simulink model "GE275103"  (R2015b)
settings: Solver=ode4  StartTime=0.0  StopTime=30  FixedStep=5e-6  RelTol=1e-3
PreLoadFcn:
  | Ts=5e-6;
values from neighbouring files (symbols this model uses):
  Cdc = 27e-3    (= 0.027)    [GE275103.m]    (also in GEWT.m)
  gear = 97    [GEWT.m]
  Jtotal = Jgen+Jtur/(gear^2)    (= 1581.65586141)    [GEWT.m]
  Ld = 10e-4    (= 0.001)    [GE275103.m]    (also in GEWT.m = 0.000248)
  Lfilter = 2e-4    (= 0.0002)    [GE275103.m]
  Lq = 10.5e-4    (= 0.00105)    [GE275103.m]    (also in GEWT.m = 0.000292)
  p = 1.225    [GE275103.m]    (also in GEWT.m)
  pgen = 2    [GE275103.m]    (also in GEWT.m = 4)
  Prated = 2750000    [GE275103.m]    (also in GEWT.m)
  R = 51.5    [GEWT.m]
  Rs = 1e-10    [GE275103.m]    (also in GEWT.m = 0.0007305)
  Vdcset = 2500    [GE275103.m]    (also in GEWT.m = 1100)
  windspeed = 10    [GEWT.m]
  winit = -160    [GEWT.m]
libraries: powerlib x17, powerlib_meascontrol x14, simulink x7
Description:
  | Copyright 2008-2013 The MathWorks, Inc.
settings Model: FPTRunName=Active  NumberOfSteps=800000  ExtModeAutoUpdateStatusClock=off  Creator=MathWorks  LastModifiedBy=Eren
settings DataIOCC: SaveFormat=Array  SignalLoggingSaveFormat=ModelDataLogs  SaveOutput=off  SignalLogging=off  SaveTime=off  SignalLoggingName=sigsOut
settings OptimizationCC: BlockReduction=off  BooleanDataType=off  ExpressionDepthLimit=2147483647  InitFltsAndDblsToZero=on
settings DebuggingCC: UnderspecifiedInitializationDetection=Classic  MergeDetectMultiDrivingBlocksExec=none  CheckExecutionContextPreStartOutputMsg=on  CheckExecutionContextRuntimeOutputMsg=on  SignalResolutionControl=TryResolveAllWithWarning  MultiTaskDSMMsg=warning  MultiTaskCondExecSysMsg=none  FcnCallInpInsideContextMsg=UseLocalSettings  StateNameClashWarn=warning
settings HardwareCC: ProdBitPerPointer=32  ProdLargestAtomicFloat=None  ProdIntDivRoundTo=Undefined  ProdEndianess=Unspecified  ProdWordSize=32  ProdHWDeviceType=32-bit Generic  TargetBitPerPointer=64  TargetLongLongMode=on  TargetIntDivRoundTo=Zero  TargetEndianess=LittleEndian  TargetWordSize=64  TargetHWDeviceType=MATLAB Host
settings GRTTargetCC: GeneratePreprocessorConditionals=Disable all  CombineOutputUpdateFcns=off  GRTInterface=on
settings ConfigComp: CovModelRefEnable=Off

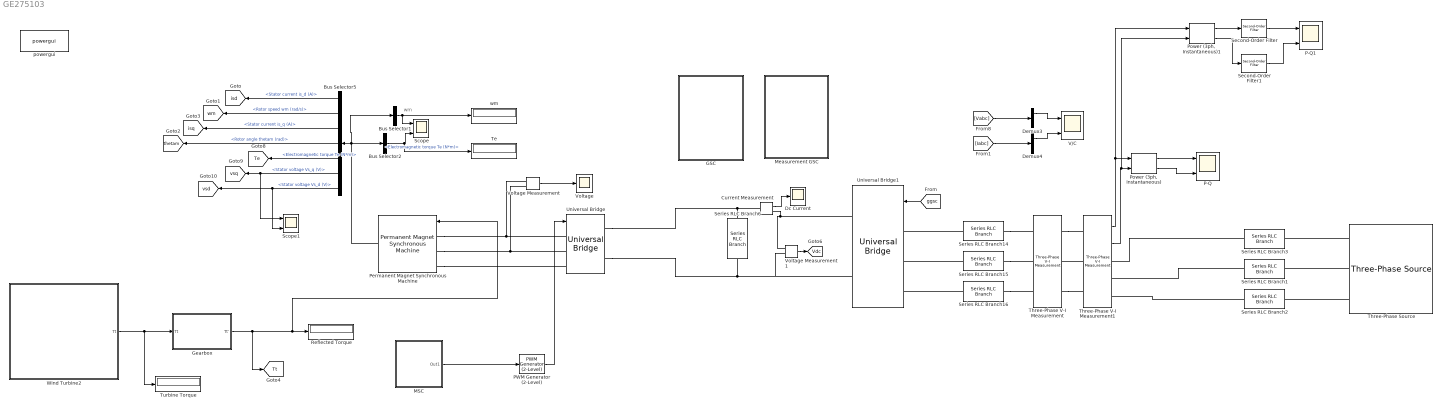
== system GE275103 ==
  note: wm
  Bus Selector1 : BusSelector  OutputSignals=Rotor speed wm (rad/s)  OutputAsBus=on
  Bus Selector2 : BusSelector  OutputSignals=Electromagnetic torque Te (N*m)
  Bus Selector5 : BusSelector  OutputSignals=Stator current is_d (A),Rotor speed wm (rad/s),Stator current is_q (A),Rotor angle thetam (rad),Electromagnetic torque Te (N*m),Stator voltage Vs_q (V),Stator voltage Vs_d (V)
  Current Measurement : powerlib/Measurements/Current Measurement  PhasorSimulation=off  OutputType=Complex  PSBequivalent=0
  Dc Current : Scope
  Demux3 : Demux  Outputs=3
  Demux4 : Demux  Outputs=3
  GSC : Subsystem
  Gearbox : Subsystem
  MSC : Subsystem
  Measurement GSC : Subsystem
  P-Q : Scope  NumInputPorts=2
  P-Q1 : Scope  NumInputPorts=2
  PWM Generator (2-Level) : powerlib_meascontrol/Pulse & Signal Generators/PWM Generator (2-Level)  ModulatorType=Three-phase bridge (6 pulses)  ModulatorMode=Unsynchronized  Fc=drivefreq  Pc=90  nF=60  MinMax="[ -1  1 ]"  SamplingTechnique=Natural  ModulatingSignals=off  m=0.8  Freq=60  Phase=0  Ts=Ts  ShowCarrierOutport=off
  Permanent Magnet Synchronous Machine : powerlib/Machines/Permanent Magnet Synchronous Machine  NbPhases=3  FluxDistribution=Sinusoidal  RotorType=Salient-pole  MechanicalLoad=Torque Tm  PresetModel=No  ShowDetailedParameters=on  MeasurementBus=off  Resistance=Rs  Inductance=8.5e-3  dqInductances=[Ld,Lq]  La=Lq  MachineConstant=Flux linkage established by magnets (V.s)  Flux=fluxlinkage  VoltageCst=1451.0395  TorqueCst=12  Flat=120  Mechanical=[Jtotal 1.349e-05 pgen 0]  PolePairs=2  InitialConditions=[winit,0, 0,0]  InitialConditions5ph=[0 0 0 0 0 0]  TsPowergui=0  TsBlock=-1  RefAngle=Aligned with phase A axis (original Park)
  "Power (3ph, Instantaneous)" : powerlib_meascontrol/Measurements/Power (3ph, Instantaneous)
  "Power (3ph, Instantaneous)1" : powerlib_meascontrol/Measurements/Power (3ph, Instantaneous)
  Reflected Torque : Display
  Scope : Scope  NumInputPorts=2
  Scope1 : Scope  NumInputPorts=2
  Second-Order Filter : powerlib_meascontrol/Filters/Second-Order Filter  FilterType=Lowpass  Fo=20  Zeta=0.707  Ts=0  Initialize=off  Vac_Init="[0,  0,  60]"  Vdc_Init=0  PlotResponse=off  FreqRange=[0, 500, 1]
  Second-Order Filter1 : powerlib_meascontrol/Filters/Second-Order Filter  FilterType=Lowpass  Fo=120  Zeta=0.707  Ts=0  Initialize=off  Vac_Init="[0,  0,  60]"  Vdc_Init=0  PlotResponse=off  FreqRange=[0, 500, 1]
  Series RLC Branch1 : powerlib/Elements/Series RLC Branch  LConnTagsString=__new0  RConnTagsString=__new0  BranchType=R  Resistance=0.001  Inductance=1e-3  SetiL0=off  InitialCurrent=0  Capacitance=1e-6  Setx0=off  InitialVoltage=0  Measurements=None
  Series RLC Branch14 : powerlib/Elements/Series RLC Branch  LConnTagsString=__new0  RConnTagsString=__new0  BranchType=L  Resistance=1  Inductance=Lfilter  SetiL0=off  InitialCurrent=0  Capacitance=1e-6  Setx0=off  InitialVoltage=0  Measurements=None
  Series RLC Branch15 : powerlib/Elements/Series RLC Branch  LConnTagsString=__new0  RConnTagsString=__new0  BranchType=L  Resistance=1  Inductance=Lfilter  SetiL0=off  InitialCurrent=0  Capacitance=1e-6  Setx0=off  InitialVoltage=0  Measurements=None
  Series RLC Branch16 : powerlib/Elements/Series RLC Branch  LConnTagsString=__new0  RConnTagsString=__new0  BranchType=L  Resistance=1  Inductance=Lfilter  SetiL0=off  InitialCurrent=0  Capacitance=1e-6  Setx0=off  InitialVoltage=0  Measurements=None
  Series RLC Branch2 : powerlib/Elements/Series RLC Branch  LConnTagsString=__new0  RConnTagsString=__new0  BranchType=R  Resistance=0.001  Inductance=1e-3  SetiL0=off  InitialCurrent=0  Capacitance=1e-6  Setx0=off  InitialVoltage=0  Measurements=None
  Series RLC Branch3 : powerlib/Elements/Series RLC Branch  LConnTagsString=__new0  RConnTagsString=__new0  BranchType=R  Resistance=0.001  Inductance=1e-3  SetiL0=off  InitialCurrent=0  Capacitance=1e-6  Setx0=off  InitialVoltage=0  Measurements=None
  Series RLC Branch6 : powerlib/Elements/Series RLC Branch  LConnTagsString=__new0  RConnTagsString=__new0  BranchType=C  Resistance=1  Inductance=1e-4  SetiL0=off  InitialCurrent=0  Capacitance=Cdc  Setx0=off  InitialVoltage=0  Measurements=None
  Te : Display
  Three-Phase V-I Measurement : powerlib/Measurements/Three-Phase V-I Measurement  VoltageMeasurement=phase-to-ground  SetLabelV=on  LabelV=Vabc  Vpu=on  VpuLL=off  CurrentMeasurement=yes  SetLabelI=on  LabelI=Iabc  Ipu=on  Pbase=2.75e6  Vbase=690  OutputType=Complex  PhasorSimulation=off  PSBequivalent=0
  Three-Phase V-I Measurement1 : powerlib/Measurements/Three-Phase V-I Measurement  VoltageMeasurement=phase-to-ground  SetLabelV=off  LabelV=Vabc  Vpu=off  VpuLL=off  CurrentMeasurement=yes  SetLabelI=off  LabelI=Iabc  Ipu=off  Pbase=2.75e6  Vbase=690  OutputType=Complex  PhasorSimulation=off  PSBequivalent=0
  Three-Phase Source : powerlib/Electrical Sources/Three-Phase Source  InternalConnection=Yg  VoltagePhases=off  Voltage=690  PhaseAngle=0  Voltage_phases=[25e3 25e3 25e3]/sqrt(3)  PhaseAngles_phases=[0 -120 +120]  Frequency=50  NonIdealSource=on  SpecifyImpedance=off  Resistance=0  Inductance=0  ShortCircuitLevel=100e6  BaseVoltage=690  XRratio=7  BusType=swing  Pref=10e3  Qref=0  Prefabc=[10e3, 10e3, 10e3]  Qrefabc=[0, 0, 0]  Qmin=-inf  Qmax=inf
  Turbine Torque : Display
  Universal Bridge : powerlib/Power Electronics/Universal Bridge  Arms=3  SnubberResistance=1e5  SnubberCapacitance=inf  Device=IGBT / Diodes  Ron=1e-3  Lon=0  ForwardVoltages="[  0  0  ]"  ForwardVoltage=0  GTOparameters=[ 10e-6 , 20e-6 ]  IGBTparameters=[ 1e-6 , 2e-6 ]  Measurements=None  Measurements_2=None  converterType=Rectifier
  Universal Bridge1 : powerlib/Power Electronics/Universal Bridge  Arms=3  SnubberResistance=1e5  SnubberCapacitance=inf  Device=IGBT / Diodes  Ron=0.00001  Lon=0  ForwardVoltages="[  0  0  ]"  ForwardVoltage=0  GTOparameters=[ 10e-6 , 20e-6 ]  IGBTparameters=[ 0 , 0 ]  Measurements=None  Measurements_2=None  converterType=Rectifier
  "V/C " : Scope  NumInputPorts=2
  Voltage : Scope
  Voltage Measurement : powerlib/Measurements/Voltage Measurement  PhasorSimulation=off  OutputType=Complex  PSBequivalent=0
  Voltage Measurement1 : powerlib/Measurements/Voltage Measurement  PhasorSimulation=off  OutputType=Complex  PSBequivalent=0
  Wind Turbine2 : Subsystem
  powergui : powerlib/powergui  Priority=2  SimulationMode=Discrete  SolverType=Tustin  SampleTime=5e-6  frequency=60  SPID=off  DisableSnubberDevices=off  DisableRonSwitches=off  DisableVfSwitches=off  SwTol=0  DisplayEquations=off  Interpol=off  ExternalGateDelay=off  methode=off  Ts=0  FunctionMessages=off  echomessages=off  HookPort=off  EnableUseOfTLC=off  x0status=blocks  frequencyindice=0  Pbase=100e6  ErrMax=1e-4  Iterations=50  UnitsV=kV  UnitsW=MW  buscounter=0  RestoreLinks=warning  ResistiveCurrentMeasurement=off  Frange=[0:2:500]  Ylog=off  Xlog=on  ShowGrid=off  save=off  variable=ZData  structure=0  ZoomFFT=on  StartTime=0.0  cycles=1  DisplayStyle=1  fundamental=60  FreqAxis=off  MaxFrequency=1000  frequencyindicesteady=1  RmsSteady=1  display=off
  wm : Display
  tag scope: Te=global, Tt=global, Vdc=global, isd=global, isq=global, thetam=global, vsd=global, vsq=global, wm=global
  wires:
  Permanent Magnet Synchronous Machine/1 -> Bus Selector5/1, Bus Selector1/1, Bus Selector2/1
  Bus Selector1/1 -> Scope/1, wm/1
  Bus Selector2/1 -> Te/1, Scope/2  "<Electromagnetic torque Te (N*m)>"
  PWM Generator (2-Level)/1 -> Universal Bridge/1
  Bus Selector5/1 -> [isd]  "<Stator current is_d (A)>"
  Bus Selector5/2 -> [wm]  "<Rotor speed wm (rad/s)>"
  Bus Selector5/4 -> [thetam]  "<Rotor angle thetam (rad)>"
  Bus Selector5/3 -> [isq]  "<Stator current is_q (A)>"
  Bus Selector5/5 -> [Te]  "<Electromagnetic torque Te (N*m)>"
  Bus Selector5/6 -> Scope1/1, [vsq]  "<Stator voltage Vs_q (V)>"
  Bus Selector5/7 -> Scope1/2, [vsd]  "<Stator voltage Vs_d (V)>"
  Wind Turbine2/1(Tt) -> Turbine Torque/1, Gearbox/1(Tt)
  Gearbox/1(Tt') -> [Tt], Permanent Magnet Synchronous Machine/1, Reflected Torque/1
  MSC/1(Out1) -> PWM Generator (2-Level)/1
  Voltage Measurement/1 -> Voltage/1
  Demux4/1 -> "V/C "/2
  Demux3/1 -> "V/C "/1
  [Vabc] -> Demux3/1
  Voltage Measurement1/1 -> [Vdc]
  [ggsc] -> Universal Bridge1/1
  "Power (3ph, Instantaneous)"/1 -> P-Q/1
  "Power (3ph, Instantaneous)"/2 -> P-Q/2
  [Iabc] -> Demux4/1
  Three-Phase V-I Measurement1/1 -> "Power (3ph, Instantaneous)1"/1, "Power (3ph, Instantaneous)"/1
  Three-Phase V-I Measurement1/2 -> "Power (3ph, Instantaneous)1"/2, "Power (3ph, Instantaneous)"/2
  Current Measurement/1 -> Dc Current/1
  "Power (3ph, Instantaneous)1"/1 -> Second-Order Filter/1
  Second-Order Filter/1 -> P-Q1/1
  "Power (3ph, Instantaneous)1"/2 -> Second-Order Filter1/1
  Second-Order Filter1/1 -> P-Q1/2
  connections:
  Permanent Magnet Synchronous Machine/LConn1 -- Voltage Measurement/LConn1 -- Universal Bridge/LConn1
  Permanent Magnet Synchronous Machine/LConn2 -- Voltage Measurement/LConn2 -- Universal Bridge/LConn2
  Permanent Magnet Synchronous Machine/LConn3 -- Universal Bridge/LConn3
  Universal Bridge/RConn1 -- Current Measurement/LConn1 -- Series RLC Branch6/LConn1
  Universal Bridge1/RConn2 -- Voltage Measurement1/LConn2 -- Universal Bridge/RConn2 -- Series RLC Branch6/RConn1
  Three-Phase V-I Measurement/RConn1 -- Three-Phase V-I Measurement1/LConn1
  Series RLC Branch1/LConn1 -- Three-Phase V-I Measurement1/RConn2
  Series RLC Branch3/LConn1 -- Three-Phase V-I Measurement1/RConn1
  Series RLC Branch15/RConn1 -- Three-Phase V-I Measurement/LConn2
  Series RLC Branch2/LConn1 -- Three-Phase V-I Measurement1/RConn3
  Three-Phase Source/RConn1 -- Series RLC Branch3/RConn1
  Series RLC Branch16/LConn1 -- Universal Bridge1/LConn3
  Series RLC Branch14/RConn1 -- Three-Phase V-I Measurement/LConn1
  Three-Phase Source/RConn3 -- Series RLC Branch2/RConn1
  Series RLC Branch16/RConn1 -- Three-Phase V-I Measurement/LConn3
  Three-Phase V-I Measurement1/LConn2 -- Three-Phase V-I Measurement/RConn2
  Three-Phase V-I Measurement/RConn3 -- Three-Phase V-I Measurement1/LConn3
  Series RLC Branch15/LConn1 -- Universal Bridge1/LConn2
  Three-Phase Source/RConn2 -- Series RLC Branch1/RConn1
  Series RLC Branch14/LConn1 -- Universal Bridge1/LConn1
  Voltage Measurement1/LConn1 -- Universal Bridge1/RConn1 -- Current Measurement/RConn1

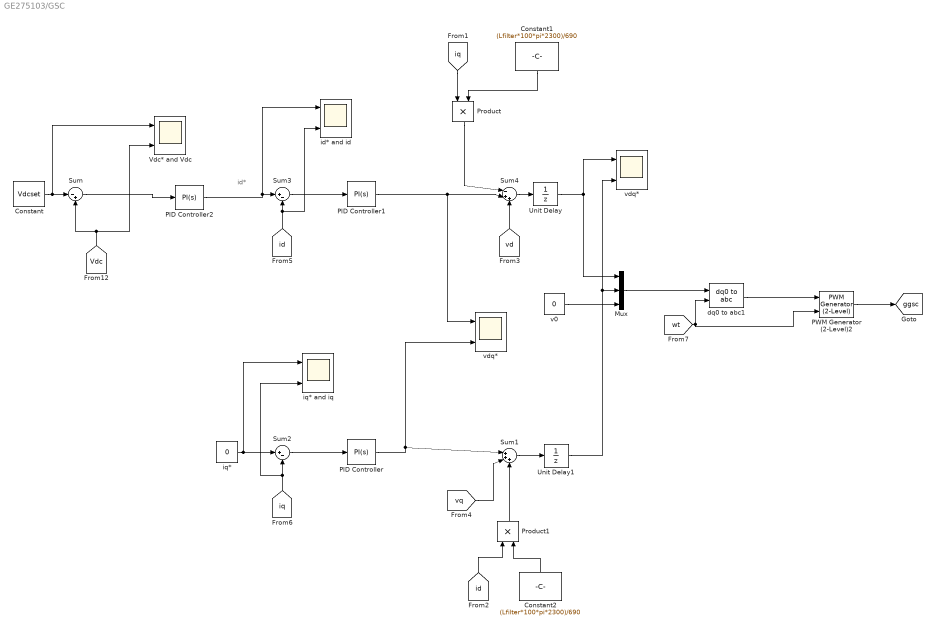
== system GE275103/GSC ==
  note: id*
  Constant : Constant  Value=Vdcset
  Constant1 : Constant  Value=(Lfilter*100*pi*2300)/690
  Constant2 : Constant  Value=(Lfilter*100*pi*2300)/690
  Mux : Mux  Inputs=3
  PID Controller : simulink/Continuous/PID Controller  Controller=PI  TimeDomain=Continuous-time  SampleTime=-1  IntegratorMethod=Forward Euler  FilterMethod=Forward Euler  Form=Parallel  UseFilter=on  ControllerParametersSource=internal  P=100  I=5  D=0  N=100  InitialConditionSource=internal  InitialConditionForIntegrator=0  InitialConditionForFilter=0  ExternalReset=none  LimitOutput=on  UpperSaturationLimit=2  LowerSaturationLimit=-2  LinearizeAsGain=on  AntiWindupMode=none  Kb=1  TrackingMode=off  Kt=1  PParamMin=[]  PParamMax=[]  IParamMin=[]  IParamMax=[]  DParamMin=[]  DParamMax=[]  NParamMin=[]  NParamMax=[]  KbParamMin=[]  KbParamMax=[]  KtParamMin=[]  KtParamMax=[]  POutMin=[]  POutMax=[]  IOutMin=[]  IOutMax=[]  DOutMin=[]  DOutMax=[]  NOutMin=[]  NOutMax=[]  KbOutMin=[]  KbOutMax=[]  KtOutMin=[]  KtOutMax=[]  IntegratorOutMin=[]  IntegratorOutMax=[]  FilterOutMin=[]  FilterOutMax=[]  SumOutMin=[]  SumOutMax=[]  SumI1OutMin=[]  SumI1OutMax=[]  SumI2OutMin=[]  SumI2OutMax=[]  SumI3OutMin=[]  SumI3OutMax=[]  SumDOutMin=[]  SumDOutMax=[]  SaturationOutMin=[]  SaturationOutMax=[]  IntegratorContinuousStateAttributes=''  IntegratorStateMustResolveToSignalObject=off  IntegratorRTWStateStorageClass=Auto  FilterContinuousStateAttributes=''  FilterStateMustResolveToSignalObject=off  FilterRTWStateStorageClass=Auto  DifferentiatorICPrevScaledInput=0  DifferentiatorOutMin=[]  DifferentiatorOutMax=[]
  PID Controller1 : simulink/Continuous/PID Controller  Controller=PI  TimeDomain=Continuous-time  SampleTime=-1  IntegratorMethod=Forward Euler  FilterMethod=Forward Euler  Form=Parallel  UseFilter=on  ControllerParametersSource=internal  P=50  I=5  D=0  N=100  InitialConditionSource=internal  InitialConditionForIntegrator=0  InitialConditionForFilter=0  ExternalReset=none  LimitOutput=on  UpperSaturationLimit=3  LowerSaturationLimit=-3  LinearizeAsGain=on  AntiWindupMode=none  Kb=1  TrackingMode=off  Kt=1  PParamMin=[]  PParamMax=[]  IParamMin=[]  IParamMax=[]  DParamMin=[]  DParamMax=[]  NParamMin=[]  NParamMax=[]  KbParamMin=[]  KbParamMax=[]  KtParamMin=[]  KtParamMax=[]  POutMin=[]  POutMax=[]  IOutMin=[]  IOutMax=[]  DOutMin=[]  DOutMax=[]  NOutMin=[]  NOutMax=[]  KbOutMin=[]  KbOutMax=[]  KtOutMin=[]  KtOutMax=[]  IntegratorOutMin=[]  IntegratorOutMax=[]  FilterOutMin=[]  FilterOutMax=[]  SumOutMin=[]  SumOutMax=[]  SumI1OutMin=[]  SumI1OutMax=[]  SumI2OutMin=[]  SumI2OutMax=[]  SumI3OutMin=[]  SumI3OutMax=[]  SumDOutMin=[]  SumDOutMax=[]  SaturationOutMin=[]  SaturationOutMax=[]  IntegratorContinuousStateAttributes=''  IntegratorStateMustResolveToSignalObject=off  IntegratorRTWStateStorageClass=Auto  FilterContinuousStateAttributes=''  FilterStateMustResolveToSignalObject=off  FilterRTWStateStorageClass=Auto  DifferentiatorICPrevScaledInput=0  DifferentiatorOutMin=[]  DifferentiatorOutMax=[]
  PID Controller2 : simulink/Continuous/PID Controller  Controller=PI  TimeDomain=Continuous-time  SampleTime=-1  IntegratorMethod=Forward Euler  FilterMethod=Forward Euler  Form=Parallel  UseFilter=on  ControllerParametersSource=internal  P=0.5  I=1.5  D=0  N=100  InitialConditionSource=internal  InitialConditionForIntegrator=0  InitialConditionForFilter=0  ExternalReset=none  LimitOutput=off  UpperSaturationLimit=inf  LowerSaturationLimit=-inf  LinearizeAsGain=on  AntiWindupMode=none  Kb=1  TrackingMode=off  Kt=1  PParamMin=[]  PParamMax=[]  IParamMin=[]  IParamMax=[]  DParamMin=[]  DParamMax=[]  NParamMin=[]  NParamMax=[]  KbParamMin=[]  KbParamMax=[]  KtParamMin=[]  KtParamMax=[]  POutMin=[]  POutMax=[]  IOutMin=[]  IOutMax=[]  DOutMin=[]  DOutMax=[]  NOutMin=[]  NOutMax=[]  KbOutMin=[]  KbOutMax=[]  KtOutMin=[]  KtOutMax=[]  IntegratorOutMin=[]  IntegratorOutMax=[]  FilterOutMin=[]  FilterOutMax=[]  SumOutMin=[]  SumOutMax=[]  SumI1OutMin=[]  SumI1OutMax=[]  SumI2OutMin=[]  SumI2OutMax=[]  SumI3OutMin=[]  SumI3OutMax=[]  SumDOutMin=[]  SumDOutMax=[]  SaturationOutMin=[]  SaturationOutMax=[]  IntegratorContinuousStateAttributes=''  IntegratorStateMustResolveToSignalObject=off  IntegratorRTWStateStorageClass=Auto  FilterContinuousStateAttributes=''  FilterStateMustResolveToSignalObject=off  FilterRTWStateStorageClass=Auto  DifferentiatorICPrevScaledInput=0  DifferentiatorOutMin=[]  DifferentiatorOutMax=[]
  PWM Generator (2-Level)2 : powerlib_meascontrol/Pulse & Signal Generators/PWM Generator (2-Level)  ModulatorType=Three-phase bridge (6 pulses)  ModulatorMode=Synchronized  Fc=50*60  Pc=90  nF=100  MinMax="[ -1  1 ]"  SamplingTechnique=Natural  ModulatingSignals=off  m=0.8  Freq=60  Phase=0  Ts=Ts  ShowCarrierOutport=off
  Product : Product
  Product1 : Product
  Sum : Sum  Inputs=|-+
  Sum1 : Sum  Inputs=|+++
  Sum2 : Sum  Inputs=|+-
  Sum3 : Sum  Inputs=|+-
  Sum4 : Sum  Inputs=|-++
  Unit Delay : UnitDelay  SampleTime=-1
  Unit Delay1 : UnitDelay  SampleTime=-1
  Vdc* and Vdc : Scope  NumInputPorts=2
  dq0 to abc1 : powerlib_meascontrol/Transformations/dq0 to abc  Alignment=90 degrees behind phase A axis
  "id* and id " : Scope  NumInputPorts=2
  iq* : Constant  Value=0
  "iq* and iq " : Scope  NumInputPorts=2
  v0 : Constant  Value=0
  vdq* : Scope  NumInputPorts=2
  "vdq* " : Scope  NumInputPorts=2
  tag scope: ggsc=global
  wires:
  PWM Generator (2-Level)2/1 -> [ggsc]
  iq*/1 -> "iq* and iq "/1, Sum2/1
  Sum3/1 -> PID Controller1/1
  PID Controller2/1 -> "id* and id "/1, Sum3/1
  [iq] -> Sum2/2, "iq* and iq "/2
  PID Controller/1 -> Sum1/1, vdq*/2
  [vq] -> Sum1/2
  [id] -> "id* and id "/2, Sum3/2
  Sum2/1 -> PID Controller/1
  PID Controller1/1 -> Sum4/2, vdq*/1
  Sum4/1 -> Unit Delay/1
  Mux/1 -> dq0 to abc1/1
  [wt] -> dq0 to abc1/2, PWM Generator (2-Level)2/2
  Sum1/1 -> Unit Delay1/1
  v0/1 -> Mux/3
  [Vdc] -> Vdc* and Vdc/2, Sum/2
  Sum/1 -> PID Controller2/1
  dq0 to abc1/1 -> PWM Generator (2-Level)2/1
  Constant/1 -> Vdc* and Vdc/1, Sum/1
  Unit Delay/1 -> Mux/1, "vdq* "/1
  Unit Delay1/1 -> "vdq* "/2, Mux/2
  [vd] -> Sum4/3
  Product/1 -> Sum4/1
  [iq] -> Product/1
  Constant1/1 -> Product/2
  Product1/1 -> Sum1/3
  [id] -> Product1/1
  Constant2/1 -> Product1/2

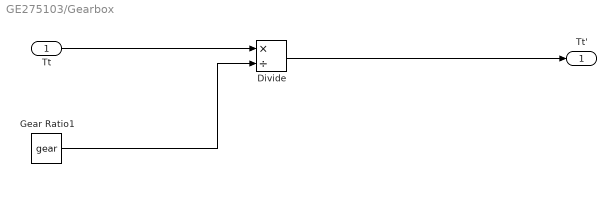
== system GE275103/Gearbox ==
  Tt : Inport
  Divide : Product  Inputs=*/
  Gear Ratio1 : Constant  Value=gear
  Tt' : Outport
  wires:
  Gear Ratio1/1 -> Divide/2
  Tt/1 -> Divide/1
  Divide/1 -> Tt'/1

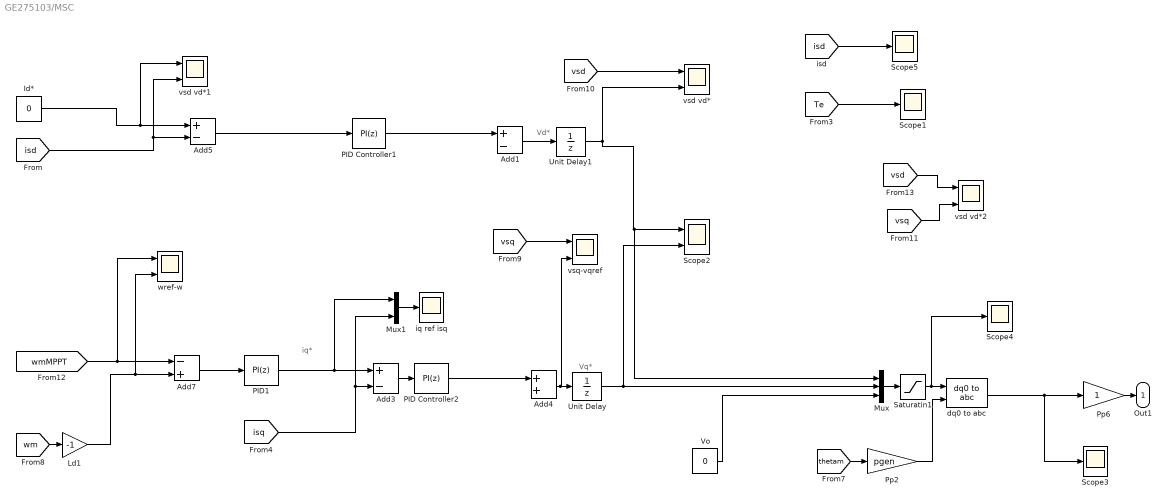
== system GE275103/MSC ==
  note: iq*
  note: Vq*
  note: Vd*
  Add1 : Sum  Inputs=+-
  Add3 : Sum  Inputs=+-
  Add4 : Sum
  Add5 : Sum  Inputs=+-
  Add7 : Sum  Inputs=-+
  Id* : Constant  Value=0
  Ld1 : Gain  Gain=-1
  Mux : Mux  Inputs=3
  Mux1 : Mux  Inputs=2
  PID Controller1 : simulink/Continuous/PID Controller  Controller=PI  TimeDomain=Discrete-time  SampleTime=-1  IntegratorMethod=Forward Euler  FilterMethod=Forward Euler  Form=Parallel  UseFilter=on  ControllerParametersSource=internal  P=20  I=2  D=0  N=100  InitialConditionSource=internal  InitialConditionForIntegrator=0  InitialConditionForFilter=0  ExternalReset=none  LimitOutput=off  UpperSaturationLimit=inf  LowerSaturationLimit=-inf  LinearizeAsGain=on  AntiWindupMode=none  Kb=1  TrackingMode=off  Kt=1  PParamMin=[]  PParamMax=[]  IParamMin=[]  IParamMax=[]  DParamMin=[]  DParamMax=[]  NParamMin=[]  NParamMax=[]  KbParamMin=[]  KbParamMax=[]  KtParamMin=[]  KtParamMax=[]  POutMin=[]  POutMax=[]  IOutMin=[]  IOutMax=[]  DOutMin=[]  DOutMax=[]  NOutMin=[]  NOutMax=[]  KbOutMin=[]  KbOutMax=[]  KtOutMin=[]  KtOutMax=[]  IntegratorOutMin=[]  IntegratorOutMax=[]  FilterOutMin=[]  FilterOutMax=[]  SumOutMin=[]  SumOutMax=[]  SumI1OutMin=[]  SumI1OutMax=[]  SumI2OutMin=[]  SumI2OutMax=[]  SumI3OutMin=[]  SumI3OutMax=[]  SumDOutMin=[]  SumDOutMax=[]  SaturationOutMin=[]  SaturationOutMax=[]  IntegratorContinuousStateAttributes=''  IntegratorStateMustResolveToSignalObject=off  IntegratorRTWStateStorageClass=Auto  FilterContinuousStateAttributes=''  FilterStateMustResolveToSignalObject=off  FilterRTWStateStorageClass=Auto  DifferentiatorICPrevScaledInput=0  DifferentiatorOutMin=[]  DifferentiatorOutMax=[]
  PID Controller2 : simulink/Continuous/PID Controller  Controller=PI  TimeDomain=Discrete-time  SampleTime=-1  IntegratorMethod=Forward Euler  FilterMethod=Forward Euler  Form=Parallel  UseFilter=on  ControllerParametersSource=internal  P=10  I=1  D=0  N=100  InitialConditionSource=internal  InitialConditionForIntegrator=0  InitialConditionForFilter=0  ExternalReset=none  LimitOutput=off  UpperSaturationLimit=inf  LowerSaturationLimit=-inf  LinearizeAsGain=on  AntiWindupMode=none  Kb=1  TrackingMode=off  Kt=1  PParamMin=[]  PParamMax=[]  IParamMin=[]  IParamMax=[]  DParamMin=[]  DParamMax=[]  NParamMin=[]  NParamMax=[]  KbParamMin=[]  KbParamMax=[]  KtParamMin=[]  KtParamMax=[]  POutMin=[]  POutMax=[]  IOutMin=[]  IOutMax=[]  DOutMin=[]  DOutMax=[]  NOutMin=[]  NOutMax=[]  KbOutMin=[]  KbOutMax=[]  KtOutMin=[]  KtOutMax=[]  IntegratorOutMin=[]  IntegratorOutMax=[]  FilterOutMin=[]  FilterOutMax=[]  SumOutMin=[]  SumOutMax=[]  SumI1OutMin=[]  SumI1OutMax=[]  SumI2OutMin=[]  SumI2OutMax=[]  SumI3OutMin=[]  SumI3OutMax=[]  SumDOutMin=[]  SumDOutMax=[]  SaturationOutMin=[]  SaturationOutMax=[]  IntegratorContinuousStateAttributes=''  IntegratorStateMustResolveToSignalObject=off  IntegratorRTWStateStorageClass=Auto  FilterContinuousStateAttributes=''  FilterStateMustResolveToSignalObject=off  FilterRTWStateStorageClass=Auto  DifferentiatorICPrevScaledInput=0  DifferentiatorOutMin=[]  DifferentiatorOutMax=[]
  PID1 : simulink/Continuous/PID Controller  Controller=PI  TimeDomain=Discrete-time  SampleTime=-1  IntegratorMethod=Forward Euler  FilterMethod=Forward Euler  Form=Parallel  UseFilter=on  ControllerParametersSource=internal  P=500  I=1500  D=0  N=100  InitialConditionSource=internal  InitialConditionForIntegrator=0  InitialConditionForFilter=0  ExternalReset=none  LimitOutput=on  UpperSaturationLimit=2300  LowerSaturationLimit=200  LinearizeAsGain=on  AntiWindupMode=none  Kb=1  TrackingMode=off  Kt=1  PParamMin=[]  PParamMax=[]  IParamMin=[]  IParamMax=[]  DParamMin=[]  DParamMax=[]  NParamMin=[]  NParamMax=[]  KbParamMin=[]  KbParamMax=[]  KtParamMin=[]  KtParamMax=[]  POutMin=[]  POutMax=[]  IOutMin=[]  IOutMax=[]  DOutMin=[]  DOutMax=[]  NOutMin=[]  NOutMax=[]  KbOutMin=[]  KbOutMax=[]  KtOutMin=[]  KtOutMax=[]  IntegratorOutMin=[]  IntegratorOutMax=[]  FilterOutMin=[]  FilterOutMax=[]  SumOutMin=[]  SumOutMax=[]  SumI1OutMin=[]  SumI1OutMax=[]  SumI2OutMin=[]  SumI2OutMax=[]  SumI3OutMin=[]  SumI3OutMax=[]  SumDOutMin=[]  SumDOutMax=[]  SaturationOutMin=[]  SaturationOutMax=[]  IntegratorContinuousStateAttributes=''  IntegratorStateMustResolveToSignalObject=off  IntegratorRTWStateStorageClass=Auto  FilterContinuousStateAttributes=''  FilterStateMustResolveToSignalObject=off  FilterRTWStateStorageClass=Auto  DifferentiatorICPrevScaledInput=0  DifferentiatorOutMin=[]  DifferentiatorOutMax=[]
  Pp2 : Gain  Gain=pgen
  Pp6 : Gain
  Saturatin1 : Saturate  UpperLimit=2000  LowerLimit=-2000
  Scope{1,3..5} (4 alike) : Scope
  Scope2 : Scope  NumInputPorts=2
  Unit Delay : UnitDelay  SampleTime=-1
  Unit Delay1 : UnitDelay  SampleTime=-1
  Vo : Constant  Value=0
  dq0 to abc : powerlib_meascontrol/Transformations/dq0 to abc  Alignment=Aligned with phase A axis
  iq ref isq : Scope
  vsd vd* : Scope  NumInputPorts=2
  vsd vd*1 : Scope  NumInputPorts=2
  vsd vd*2 : Scope  NumInputPorts=2
  vsq-vqref : Scope  NumInputPorts=2
  wref-w : Scope  NumInputPorts=2
  Out1 : Outport
  wires:
  dq0 to abc/1 -> Pp6/1, Scope3/1
  Mux/1 -> Saturatin1/1
  Vo/1 -> Mux/3
  Add3/1 -> PID Controller2/1
  Add5/1 -> PID Controller1/1
  PID Controller1/1 -> Add1/1
  Add1/1 -> Unit Delay1/1
  [thetam] -> Pp2/1
  Pp2/1 -> dq0 to abc/2
  [vsq] -> vsq-vqref/1
  [vsd] -> vsd vd*/1
  Mux1/1 -> iq ref isq/1
  [isd] -> Scope5/1
  [Te] -> Scope1/1
  Saturatin1/1 -> Scope4/1, dq0 to abc/1
  Add4/1 -> vsq-vqref/2, Unit Delay/1
  Add7/1 -> PID1/1
  [wm] -> Ld1/1
  Ld1/1 -> Add7/2, wref-w/2
  [wmMPPT] -> Add7/1, wref-w/1
  Id*/1 -> vsd vd*1/1, Add5/1
  [isd] -> vsd vd*1/2, Add5/2
  [isq] -> Mux1/2, Add3/2
  Pp6/1 -> Out1/1
  PID1/1 -> Mux1/1, Add3/1
  [vsd] -> vsd vd*2/1
  [vsq] -> vsd vd*2/2
  PID Controller2/1 -> Add4/1
  Unit Delay/1 -> Scope2/2, Mux/2
  Unit Delay1/1 -> Mux/1, Scope2/1, vsd vd*/2

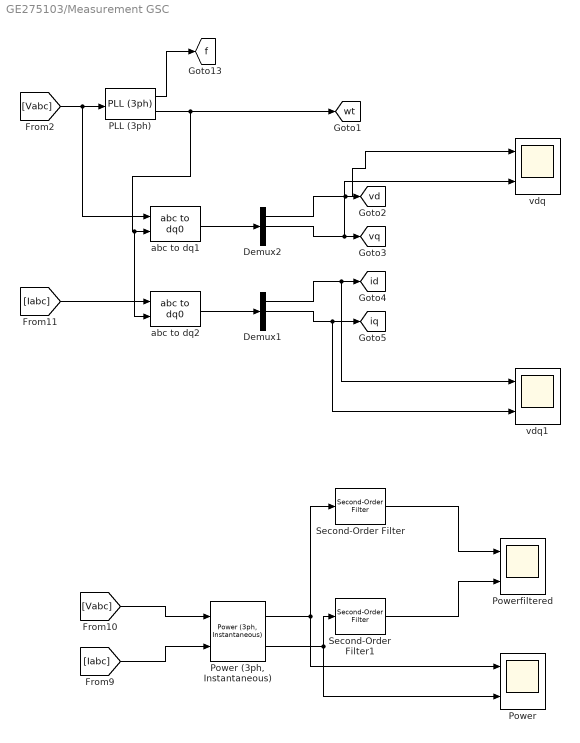
== system GE275103/Measurement GSC ==
  Demux1 : Demux  Outputs=3
  Demux2 : Demux  Outputs=3
  PLL (3ph) : powerlib_meascontrol/PLL/PLL (3ph)  Fmin=45  Par_Init=[0, 50]  ParK=[180, 3200, 1]  TcD=1e-4  MaxRateChangeFreq=12  FilterCutOffFreq=25  Ts=Ts  AGC=on
  Power : Scope  NumInputPorts=2
  "Power (3ph, Instantaneous)" : powerlib_meascontrol/Measurements/Power (3ph, Instantaneous)
  "Powerfiltered " : Scope  NumInputPorts=2
  Second-Order Filter : powerlib_meascontrol/Filters/Second-Order Filter  FilterType=Lowpass  Fo=50  Zeta=0.707  Ts=Ts  Initialize=off  Vac_Init="[0,  0,  60]"  Vdc_Init=0  PlotResponse=off  FreqRange=[0, 500, 1]
  Second-Order Filter1 : powerlib_meascontrol/Filters/Second-Order Filter  FilterType=Lowpass  Fo=100  Zeta=0.707  Ts=0  Initialize=off  Vac_Init="[0,  0,  60]"  Vdc_Init=0  PlotResponse=off  FreqRange=[0, 500, 1]
  abc to dq1 : powerlib_meascontrol/Transformations/abc to dq0  Alignment=90 degrees behind phase A axis
  abc to dq2 : powerlib_meascontrol/Transformations/abc to dq0  Alignment=90 degrees behind phase A axis
  vdq : Scope  NumInputPorts=2
  vdq1 : Scope  NumInputPorts=2
  tag scope: f=global, id=global, iq=global, vd=global, vq=global, wt=global
  wires:
  PLL (3ph)/1 -> [f]
  [Vabc] -> abc to dq1/1, PLL (3ph)/1
  PLL (3ph)/2 -> abc to dq2/2, abc to dq1/2, [wt]
  [Iabc] -> abc to dq2/1
  Demux2/1 -> vdq/1, [vd]
  Demux2/2 -> vdq/2, [vq]
  Demux1/1 -> vdq1/1, [id]
  Demux1/2 -> vdq1/2, [iq]
  abc to dq1/1 -> Demux2/1
  abc to dq2/1 -> Demux1/1
  "Power (3ph, Instantaneous)"/1 -> Power/1, Second-Order Filter/1
  "Power (3ph, Instantaneous)"/2 -> Power/2, Second-Order Filter1/1
  Second-Order Filter1/1 -> "Powerfiltered "/2
  Second-Order Filter/1 -> "Powerfiltered "/1
  [Vabc] -> "Power (3ph, Instantaneous)"/1
  [Iabc] -> "Power (3ph, Instantaneous)"/2

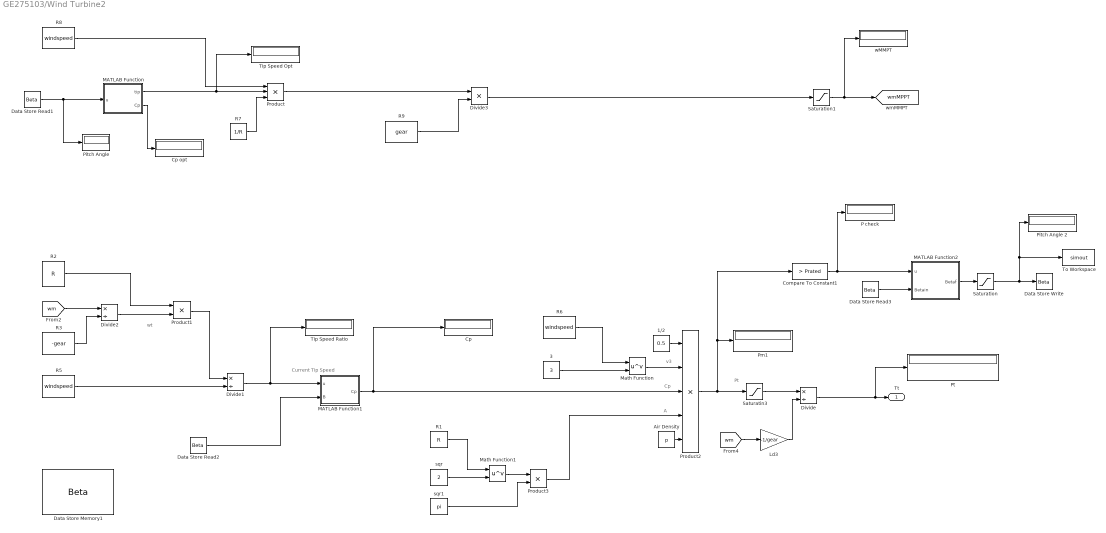
== system GE275103/Wind Turbine2 ==
  note: Pt
  note: v3
  note: Cp
  note: A
  note: wt
  note: Current Tip Speed
  1/2 : Constant  Value=0.5
  3 : Constant  Value=3
  Air Density : Constant  Value=p
  Compare To Constant1 : simulink/Logic and Bit Operations/Compare To Constant  relop=>  const=Prated  OutDataTypeStr=boolean
  Cp : Display
  Cp opt : Display
  Data Store Memory1 : DataStoreMemory  DataStoreName=Beta  ReadBeforeWriteMsg=warning  WriteAfterWriteMsg=warning  WriteAfterReadMsg=warning  OutMin=[0]  OutMax=[90]
  Data Store Read1 : DataStoreRead  DataStoreName=Beta  SampleTime=Ts
  Data Store Read2 : DataStoreRead  DataStoreName=Beta  SampleTime=Ts
  Data Store Read3 : DataStoreRead  DataStoreName=Beta  SampleTime=Ts
  Data Store Write : DataStoreWrite  DataStoreName=Beta
  Divide : Product  Inputs=*/
  Divide1 : Product  Inputs=*/
  Divide2 : Product  Inputs=*/
  Divide3 : Product  Inputs=**
  Ld3 : Gain  Gain=-1/gear
  MATLAB Function : MATLAB Function  TreatAsAtomicUnit=on
  MATLAB Function1 : MATLAB Function  TreatAsAtomicUnit=on
  MATLAB Function2 : MATLAB Function  TreatAsAtomicUnit=on
  Math Function : Math  Operator=pow  SaturateOnIntegerOverflow=on
  Math Function1 : Math  Operator=pow  SaturateOnIntegerOverflow=on
  P check : Display
  "Pitch Angle " : Display
  Pitch Angle 2 : Display
  Pm1 : Display
  Product : Product  Inputs=3
  Product1 : Product
  Product2 : Product  Inputs=5
  Product3 : Product
  Pt : Display
  R1 : Constant  Value=R
  R2 : Constant  Value=R
  R3 : Constant  Value=-gear
  R5 : Constant  Value=windspeed
  R6 : Constant  Value=windspeed
  R7 : Constant  Value=1/R
  R8 : Constant  Value=windspeed
  R9 : Constant  Value=gear
  Saturatin3 : Saturate  UpperLimit=2.75e6  LowerLimit=1e6
  Saturation : Saturate  UpperLimit=90  LowerLimit=0
  Saturation1 : Saturate  UpperLimit=181.68  LowerLimit=0
  "Tip Speed Opt " : Display
  "Tip Speed Ratio " : Display
  To Workspace : ToWorkspace  VariableName=simout  SaveFormat=Timeseries  SampleTime=-1
  sqr : Constant  Value=2
  sqr1 : Constant  Value=pi
  "wMMPT " : Display
  Tt : Outport
  tag scope: wmMPPT=global
  wires:
  Air Density/1 -> Product2/5
  1/2/1 -> Product2/1
  Product3/1 -> Product2/4
  Math Function1/1 -> Product3/1
  sqr1/1 -> Product3/2
  [wm] -> Ld3/1
  Math Function/1 -> Product2/2
  sqr/1 -> Math Function1/2
  R1/1 -> Math Function1/1
  Product2/1 -> Saturatin3/1, Compare To Constant1/1, Pm1/1
  3/1 -> Math Function/2
  R2/1 -> Product1/1
  [wm] -> Divide2/1
  Product1/1 -> Divide1/1
  R5/1 -> Divide1/2
  Divide1/1 -> MATLAB Function1/1(u), "Tip Speed Ratio "/1
  Divide2/1 -> Product1/2
  Ld3/1 -> Divide/2
  MATLAB Function1/1(Cp) -> Product2/3, Cp/1
  R3/1 -> Divide2/2
  R6/1 -> Math Function/1
  MATLAB Function/1(tip) -> "Tip Speed Opt "/1, Product/2
  R7/1 -> Product/3
  R8/1 -> Product/1
  Product/1 -> Divide3/1
  R9/1 -> Divide3/2
  MATLAB Function/2(Cp) -> Cp opt/1
  Divide3/1 -> Saturation1/1
  Data Store Read3/1 -> MATLAB Function2/2(Betain)
  Data Store Read2/1 -> MATLAB Function1/2(B)
  Data Store Read1/1 -> "Pitch Angle "/1, MATLAB Function/1(u)
  MATLAB Function2/1(Betaf) -> Saturation/1
  Compare To Constant1/1 -> MATLAB Function2/1(u), P check/1
  Saturation/1 -> To Workspace/1, Pitch Angle 2/1, Data Store Write/1
  Saturation1/1 -> "wMMPT "/1, [wmMPPT]
  Divide/1 -> Pt/1, Tt/1
  Saturatin3/1 -> Divide/1

== matlab function GE275103/Wind Turbine2/MATLAB Function ==
  data: u input; tip output; Cp output
function [tip,Cp]= fcn(u)

c1 = 0.5176;
c2 = 116;
c3 = 0.4;
c4 = 5;
c5 = 21;
c6 = 0.0068;
B=0;
for i = 0.1:0.1:15
    
li = 1/((1/(i+0.08*u))-(0.035/(u^3+1)));
A = c1*((c2/li-c3*u-c4)*exp(-c5/li))+c6*i ;%#codegen

    if A < B
    lopt = i;
    break
    else 
    B = A;
    end
end
tip = i;
Cp = c1*((c2/li-c3*u-c4)*exp(-c5/li))+c6*i;
end

== matlab function GE275103/Wind Turbine2/MATLAB Function1 ==
  data: u input; B input; Cp output
function Cp = fcn(u,B)

c1 = 0.5176;
c2 = 116;
c3 = 0.4; 
c4 = 5;
c5 = 21;
c6 = 0.0068;

i =u;

li = 1/((1/(i+0.08*B))-(0.035/(B^3+1)));

Cp = c1*((c2/li-c3*B-c4)*exp(-c5/li))+c6*i;

end

== matlab function GE275103/Wind Turbine2/MATLAB Function2 ==
  data: u input; Betaf output; Betain input
function Betaf  = fcn(u,Betain)

    if u ==1
    Betaf = Betain+0.01;
    else  

    Betaf = Betain-0.01;
    end
 
    
    
end
